simulink model "relay_template"  (R2015a)
settings: Solver=ode1  SolverMode=SingleTasking  StartTime=0.0  StopTime=20  FixedStep=0.01  RelTol=1e-3
values from neighbouring files (symbols this model uses):
  d = 2.5    [exp9.m]    (also in exp9_ptestes.m)
  epsulon = 0    [exp9.m]    (also in exp9_ptestes.m)
  KP = 0.6*Ku    (= 6.62800387681)    [exp9.m]    (also in exp9_ptestes.m = 2.42800387681)
  N = 10    [exp9.m]    (also in exp9_ptestes.m)
  Td = Tu/8    (= 0.0875)    [exp9.m]    (also in exp9_ptestes.m = 0.1275)
  Ti = Tu/2    (= 0.35)    [exp9.m]    (also in exp9_ptestes.m = 0.5)
settings Model: CovSFcnEnable=off  Creator=rpm  LastModifiedBy=sasuk
settings DataIOCC: LimitDataPoints=off  SignalLoggingSaveFormat=ModelDataLogs  SaveOutput=off  SignalLogging=off  TimeSaveName=t
settings OptimizationCC: ExpressionDepthLimit=2147483647  InitFltsAndDblsToZero=on
settings DebuggingCC: UnderspecifiedInitializationDetection=Classic  MergeDetectMultiDrivingBlocksExec=none  FcnCallInpInsideContextMsg=UseLocalSettings  StateNameClashWarn=warning
settings GRTTargetCC: CombineOutputUpdateFcns=off  GRTInterface=on

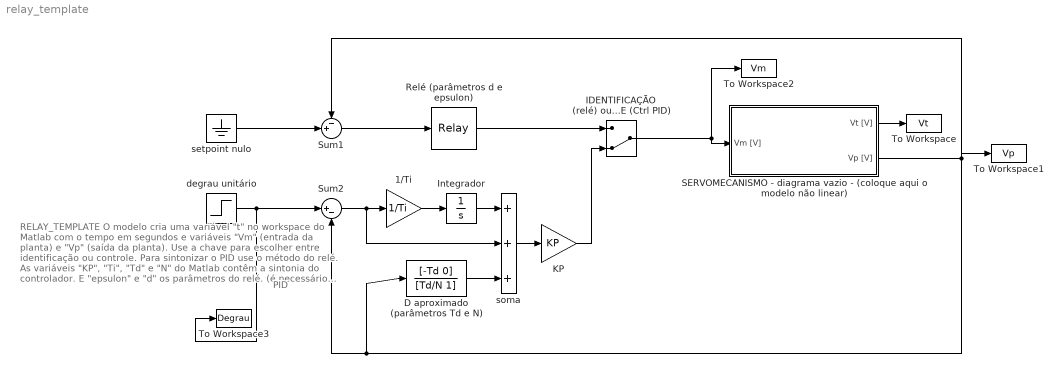
== system relay_template ==
  note: RELAY_TEMPLATE
      |
      | O modelo cria uma variável "t" no workspace
      | do Matlab com o tempo em segundos e variáveis
      | "Vm" (entrada da planta) e "Vp" (saída da planta).
      |
      | Use a chave para escolher entre identificação
      | ou controle.
      |
      | Para sintonizar o PID use o método do relé.
      |
      | As variáveis "KP", "Ti", "Td" e "N" do Matlab
      | contêm a sintonia do controlador. E "epsulon" e "d"
      | os parâmetros do relé.
      | (é necessário criá-las para que não haja
      | erros na simulação, mesmo se não
      | forem usadas).
      |
      | IMPORTANTE: Caso o sistema não saia do
      | equilíbrio e entre expontaneamente em oscilação
      | para alguma configuração de "d" e "epsulon",
      | use uma condição inicial diferente de zero para a
      | posição (no servomecanismo real o ruído de
      | medida em geral já é suficiente para
      | provocar oscilação).
  note: PID
  1/Ti : Gain  Gain=1/Ti
  D aproximado (parâmetros Td e N) : TransferFcn  Numerator=[-Td 0]  Denominator=[Td/N 1]
  IDENTIFICAÇÃO (relé) ou CONTROLE (Ctrl PID) : ManualSwitch  CurrentSetting=0
  Integrador : Integrator
  KP : Gain  Gain=KP
  Relé (parâmetros d e epsulon) : Relay  OnSwitchValue=epsulon  OffSwitchValue=-epsulon  OnOutputValue=d  OffOutputValue=-d
  SERVOMECANISMO - diagrama vazio - (coloque aqui o modelo não linear) : Subsystem
  Sum1 : Sum  Inputs=-+|
  Sum2 : Sum  Inputs=|+-
  To Workspace : ToWorkspace  VariableName=Vt  SampleTime=-1
  To Workspace1 : ToWorkspace  VariableName=Vp  SampleTime=-1
  To Workspace2 : ToWorkspace  VariableName=Vm  SampleTime=-1
  To Workspace3 : ToWorkspace  VariableName=Degrau  SampleTime=-1
  degrau unitário : Step  After=1.59  SampleTime=0
  setpoint nulo : Ground
  soma : Sum  Inputs=+++
  wires:
  IDENTIFICAÇÃO (relé) ou CONTROLE (Ctrl PID)/1 -> To Workspace2/1, SERVOMECANISMO - diagrama vazio - (coloque aqui o modelo não linear)/1(Vm [V])
  degrau unitário/1 -> To Workspace3/1, Sum2/1
  KP/1 -> IDENTIFICAÇÃO (relé) ou CONTROLE (Ctrl PID)/2
  soma/1 -> KP/1
  Integrador/1 -> soma/1
  1/Ti/1 -> Integrador/1
  Sum2/1 -> 1/Ti/1, soma/2
  Relé (parâmetros d e epsulon)/1 -> IDENTIFICAÇÃO (relé) ou CONTROLE (Ctrl PID)/1
  Sum1/1 -> Relé (parâmetros d e epsulon)/1
  setpoint nulo/1 -> Sum1/2
  SERVOMECANISMO - diagrama vazio - (coloque aqui o modelo não linear)/2(Vp [V]) -> Sum2/2, D aproximado (parâmetros Td e N)/1, Sum1/1, To Workspace1/1
  SERVOMECANISMO - diagrama vazio - (coloque aqui o modelo não linear)/1(Vt [V]) -> To Workspace/1
  D aproximado (parâmetros Td e N)/1 -> soma/3

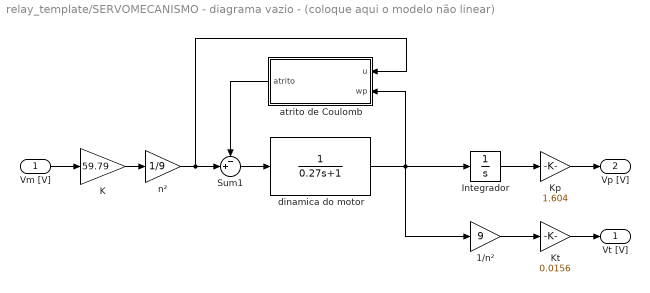
== system relay_template/SERVOMECANISMO - diagrama vazio - (coloque aqui o modelo não linear) ==
  Vm [V] : Inport
  1/n² : Gain  Gain=9
  Integrador : Integrator
  K : Gain  Gain=59.79
  Kp : Gain  Gain=1.604
  Kt : Gain  Gain=0.0156
  Sum1 : Sum  Inputs=-+|
  atrito de Coulomb : Subsystem  mask{phi=1.2088}
      mask Display: fprintf('phi = %3.1f', phi)
  dinamica do motor : TransferFcn  Denominator=[0.27 1]
  n² : Gain  Gain=1/9
  Vt [V] : Outport
  Vp [V] : Outport  Port=2
  wires:
  dinamica do motor/1 -> atrito de Coulomb/2(wp), 1/n²/1, Integrador/1
  Integrador/1 -> Kp/1
  Kt/1 -> Vt [V]/1
  Kp/1 -> Vp [V]/1
  K/1 -> n²/1
  n²/1 -> atrito de Coulomb/1(u), Sum1/2
  atrito de Coulomb/1(atrito) -> Sum1/1
  Sum1/1 -> dinamica do motor/1
  1/n²/1 -> Kt/1
  Vm [V]/1 -> K/1

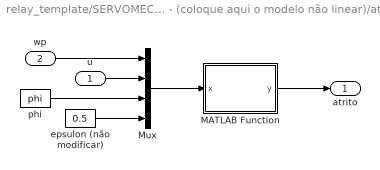
== system relay_template/SERVOMECANISMO - diagrama vazio - (coloque aqui o modelo não linear)/atrito de Coulomb ==
  u : Inport
  wp : Inport  Port=2
  MATLAB Function : MATLAB Function  TreatAsAtomicUnit=on
  Mux : Mux
  epsulon (não modificar) : Constant  Value=0.5
  phi : Constant  Value=phi
  atrito : Outport
  wires:
  u/1 -> Mux/2
  phi/1 -> Mux/3
  MATLAB Function/1(y) -> atrito/1
  wp/1 -> Mux/1
  epsulon (não modificar)/1 -> Mux/4
  Mux/1 -> MATLAB Function/1(x)

== matlab function relay_template/SERVOMECANISMO - diagrama vazio - (coloque aqui o modelo não linear)/atrito de Coulomb/MATLAB Function ==
  data: x input size=4; y output size=1
function y = nl_coulomb(x)
% Atrito de Coulomb
% Para uso de nl_template.mdl

wp  = x(1); 
u   = x(2); 
phi = x(3); 
epsulon = x(4);

y = 0;

if wp > epsulon
    y = phi;
elseif wp < -epsulon
    y = -phi;
elseif wp >= 0
    y = min(phi,abs(u));
elseif wp < 0
    y = max(-phi,-abs(u));
end
